simulink model "simulator"  (R2025b)
settings: Solver=ode3  StartTime=0.0  StopTime=30  FixedStep=1e-3  RelTol=1e-3
settings Model: Creator=ateveraz  LastModifiedBy=ateveraz

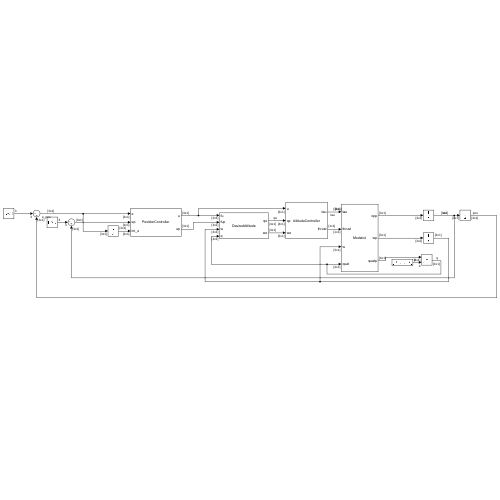
[thumbnail: Simulink's stored preview of the top-level diagram]
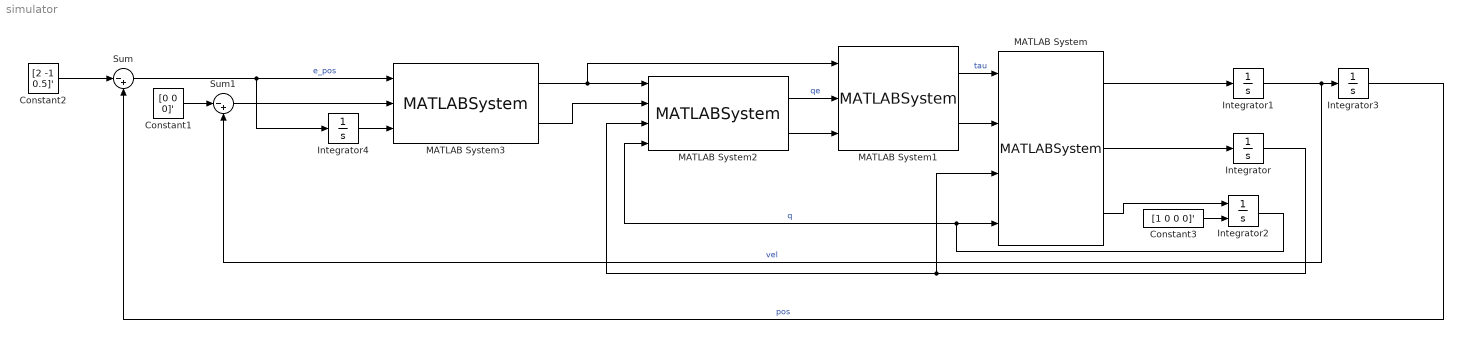
== system simulator ==
  Constant1 : Constant  Value=[0 0 0]'
  Constant2 : Constant  Value=[2 -1 0.5]'
  Constant3 : Constant  Value=[1 0 0 0]'
  Integrator : Integrator  InitialCondition=[0 0 0]'
  Integrator1 : Integrator  InitialCondition=[0 0 0]'
  Integrator2 : Integrator  InitialConditionSource=external  InitialCondition=[1 0 0 0]'
  Integrator3 : Integrator  InitialCondition=[1 1 1]'
  Integrator4 : Integrator  InitialCondition=[0 0 0]'
  MATLAB System : MATLABSystem  System=Modelx4  linear_position=[ 1; 1; 1]  linear_velocity=[ 0; 0; 0 ]  quaternion=[ 1, 0, 0, 0 ]'  angular_velocity=[ 0; 0; 0 ]  euler_angles=[ 0, 0, 0 ]  SimulateUsing=Code generation
      mask Type: Modelx4
  MATLAB System1 : MATLABSystem  System=AttitudeController  Kd=2.0  beta=0.5  gamma=1.0  rho=5.0  SimulateUsing=Code generation
      mask Type: AttitudeController
  MATLAB System2 : MATLABSystem  System=DesiredAttitude  SimulateUsing=Code generation
      mask Type: DesiredAttitude
  MATLAB System3 : MATLABSystem  System=PositionController  Kp=3  Kd=2  Ki=1  SimulateUsing=Code generation
      mask Type: PositionController
  Sum : Sum  Inputs=|-+
  Sum1 : Sum  Inputs=|-+
  wires:
  MATLAB System/2 -> Integrator/1
  MATLAB System/1 -> Integrator1/1
  Integrator/1 -> MATLAB System/3, MATLAB System2/3
  MATLAB System/3 -> Integrator2/1
  Integrator2/1 -> MATLAB System2/4, MATLAB System/4  "q"
  Constant3/1 -> Integrator2/2
  Integrator1/1 -> Sum1/2, Integrator3/1  "vel"
  Integrator3/1 -> Sum/2  "pos"
  MATLAB System1/1 -> MATLAB System/1  "tau"
  Constant1/1 -> Sum1/1
  Constant2/1 -> Sum/1
  MATLAB System2/1 -> MATLAB System1/2  "qe"
  MATLAB System2/2 -> MATLAB System1/3
  MATLAB System3/1 -> MATLAB System1/1, MATLAB System2/1
  MATLAB System1/2 -> MATLAB System/2
  MATLAB System3/2 -> MATLAB System2/2
  Sum/1 -> Integrator4/1, MATLAB System3/1  "e_pos"
  Sum1/1 -> MATLAB System3/2
  Integrator4/1 -> MATLAB System3/3
